simulink model "Eem_StMac_Prj"  (R2013b)
settings: Solver=FixedStepDiscrete  StartTime=0.0  StopTime=inf  FixedStep=0.001  RelTol=1e-3
PreLoadFcn:
  | load('Eem_StMac_Sim_DataSpec.mat')
model workspace (MAT data in the model file):
  java : class17 (value not decoded)
  MCOS : class17 (value not decoded)
undefined symbols (not defined in the file): process, ProcessTrigger_Lib
libraries: Variable_Lib x21, Efx_Library x17, Parameter_Lib x16, DSM_Library x9, DeltaTime_Lib x2, SYC_Library x1, DGS_Misc_Lib x1
(part 2 of 2)

== stateflow chart Eem_StMac_Prj/Eem_StMac/Component_Functionality/Proc_10ms/EemStrtupShdwn_SF ==
  note: Eem_stAct shows present state for simulation
  state Init_Mode
    state Eem_stAct_1
      entry:
      Eem_stAct = 1; ...
      Eem_tiStEx = 0;
      //***********************************
      Eem_stDesBms = 0; ...
      Eem_stDesPt = 1; ...
      Eem_stDesDcdc = 0; ...
      //***********************************
  note: Waiting for Transition from Car, Startup Demand from "above"
  note: Startwish by driver
  state Init_Mode_BattOn_BRMOn
    state Eem_stAct_5
      entry:
      Eem_stAct = 5; ...
      //***********************************
      // nothing to do
      // waiting BRM/battery ECUs to be switched on
      //***********************************
  note: power on: batttery ECU and BRM ECU
  note: Batt pre run test finished and
      | BRM inittest with 14 V ready and
      | DCDC preruntest finished
  state Startup_Mode
    during:
    Eem_tiStEx=Eem_tiStEx +dT;
    note: Battery, BRM, DCDC: be ready for PreCharge !
    state Eem_stAct_10
      entry:
      Eem_tiStEx =0;
      //***********************************
      // no change
      //***********************************
      Eem_stAct =10;
      note: Start Initialisation
    note: Battery, BRM, DCDC are ready for PreCharge
    note: Init of all components finished,
        | voltage level for successful  PreCharge
        | is reached
    note: Init of all components finished,
        | voltage level for successful  PreCharge
        | is reached
    note: Precharge with DCDC-converter
    state Eem_stAct_16
      entry:
      //*************************************
      Eem_stDesBms = 5; ...
      //**************************************
      Eem_stAct = 16;
      note: Init finished
    state Eem_stAct_14
      entry:
      //*****************************
      Eem_stDesDcdc = 3; ...
      //*****************************
      Eem_stAct = 14;
    note: PreCharge with Battery
    state Eem_stAct_12
      entry:
      //******************************
      Eem_stDesBms = 3; ...
      //****************************
      Eem_stAct = 12;
    note: PreCharge finished
        |  => Battery has to close main relais
    note: Mainrelais is closed
    state Eem_stAct_20
      entry:
      //**********************************
      Eem_stDesPt = 5; ...
      Eem_stDesDcdc = 5; ...
      //*********************************
      Eem_stAct = 20;
      note: Idle requested
    note: components in idle
    state Eem_stAct_30
      entry:
      //**********************************
      Eem_stDesPt = 6; ....
      //*********************************
      Eem_stAct = 30;
      note: PTr be boss
    (default) -> Eem_stAct_10
    (junction 153) -> Eem_stAct_14 [order 1] : [PRECOPT_SC ==0]
    Eem_stAct_10 -> (junction 153)
    (junction 153) -> Eem_stAct_12 [order 2] : [PRECOPT_SC >=1]
    Eem_stAct_12 -> Eem_stAct_16 : [Mvb_stOperModAct == 4 && ...
        | abs(Mvb_uAct - Dcdc_uMvAct) < Eem_uDifPtdPrec_C && ...
        | abs(Mvb_uAct - ElM_uAct) < Eem_uDifPtdPrec_C && ...
        | abs(Mvb_iAct) < Eem_iMinNcsryCntctr_C ]
    Eem_stAct_14 -> Eem_stAct_16 : [Dcdc_stOperModAct == 3 && ...
        | abs(Mvb_uAct - Dcdc_uMvAct) < Eem_uDifPtdPrec_C && ...
        | abs(Mvb_uAct - ElM_uAct) < Eem_uDifPtdPrec_C && ...
        | abs(Dcdc_iMvAct) < Eem_iMinNcsryCntctr_C]
    Eem_stAct_16 -> Eem_stAct_20 : [Mvb_stOperModAct == 5]
    Eem_stAct_20 -> Eem_stAct_30 : [ElM_stOperModAct == 5 && ...
        |  Dcdc_stOperModAct == 5 ]
  note: Pre Charging and closing of battery connectors
  state Service Modes [group]
    note: Not yet used
  note: BRM has taken over control
  state Normal_Mode
    entry:
    Eem_tiStEx=0;
    (history)
    note: PTr has torque control
    note: BRS-Normal Operation mode
        | with DCDC in forward mode
    note: BRS-Normal Operation mode
        | with DCDC in reverse mode
    note: no BRM start
    note: BRM start
    state Eem_stAct_46
      entry:
      //*****************************
      Eem_stDesDcdc = 8;
      //*****************************
      Eem_stAct = 46;
      note: no ICE-start with BRM ->
          | start with 12-V-starter
    state Eem_stAct_47
      entry:
      //***************************
      Eem_stDesDcdc = 9;
      //****************************
      Eem_stAct = 47;
      note: ICE-start with BRM
    (default) -> Eem_stAct_46
    Eem_stAct_47 -> Eem_stAct_46 : [ElM_stOperModAct != 11]
    Eem_stAct_46 -> Eem_stAct_47 : [ElM_stOperModAct == 11]
  state Backup_Modes
    entry:
    Eem_tiStEx = 0;
    note: default transition leads to backupmode 600
    note: "Battery off"
    note: "Battery off with
        | communication loss"
    note: "Generator limitted"
    note: "BRM off"
    note: "DCDC off"
    note: "DCDC off with
        |  commincation loss"
    note: "all off after load reduction
    note: "Emergency off" (even under load)
    note: BRM works as Generator with limitted load
    note: BRM voltage controlled and DCDC in forwar,
        |  battery has to disconnect by itself
    note: shorttime switch off of Dcdc and BRM
    note: BRM, DCDC and battery off
    note: BRM voltagecontrolled,
        | DCDC in forward mode
    note: BRM off
    note: Switch off DCDC-Converter
    state Eem_stAct_196
      entry:
      //**************************
      Eem_stDesPt = 5; ...
      Eem_stDesDcdc = 5; ...
      //*************************
      Eem_stAct=196;
      during:
      Eem_tiStEx = Eem_tiStEx + dT;
    state Eem_stAct_700
      entry:
      //**************************
      Eem_stDesBms = 14; ...
      Eem_stDesPt = 13; ...
      Eem_stDesDcdc = 13; ...
      //***************************
      Eem_stAct=700;
    state Eem_stAct_550
      entry:
      //****************************
      //* nothing **/
      //*****************************
      Eem_stAct=550;
    state Eem_stAct_598
      entry:
      //****************************
      Eem_stDesPt = 5; ...
      Eem_stDesDcdc = 5; ...
      //*****************************
      Eem_stAct=598;
      during:
      Eem_tiStEx = Eem_tiStEx + dT;
    state Eem_stAct_300
      entry:
      //***********************
      Eem_stDesPt = 7; ...
      Eem_stDesDcdc = 8; ...
      //***********************
      Eem_stAct=300;
    state Eem_stAct_400
      entry:
      //************************
      Eem_stDesPt = 13; ...
      //************************
      Eem_stAct=400;
    state Eem_stAct_250
      entry:
      //**************************
      Eem_stDesPt = 7; ...
      Eem_stDesDcdc = 8; ...
      //*************************
      Eem_stAct=250;
    state Eem_stAct_500
      entry:
      //****************************
      Eem_stDesDcdc = 13; ...
      //*****************************
      Eem_stAct=500;
    note: condition for "no currentflow over battery contactors"
    note: !! fail save state !!
    note: condition for "no currentflow over battery contactors"
    state Eem_stAct_198
      entry:
      //*****************************
      Eem_stDesBms = 13; ...
      //*****************************
      Eem_stAct = 198;
      during:
      Eem_tiStEx = Eem_tiStEx + dT;
    note: disconnection of 48V battery
    state Eem_stAct_600
      entry:
      //*****************************
      Eem_stDesBms = 13; ...
      Eem_stDesPt = 13; ...
      Eem_stDesDcdc = 13; ...
      //*****************************
      Eem_stAct = 600;
    note: condition for "MV grid is down"
    state Eem_stAct_200
      entry:
      Eem_tiStEx =0 ;...
      //*****************************
      Eem_stDesPt = 7; ...
      Eem_stDesDcdc = 8; ...
      //****************************
      Eem_stAct = 200;
    note: BRM voltage controlled
        | DCDC in forward mode
    note: battery is disconnected
    (junction 545) -> Eem_stAct_700 [order 1] : [Eem_stDesBkup == 700]
    (default) -> (junction 545)
    (junction 545) -> Eem_stAct_598 [order 8]
    (junction 545) -> Eem_stAct_196 [order 5] : [Eem_stDesBkup == 200]
    (junction 545) -> Eem_stAct_550 [order 7] : [Eem_stDesBkup == 550]
    (junction 545) -> Eem_stAct_250 [order 6] : [Eem_stDesBkup == 250]
    (junction 545) -> Eem_stAct_500 [order 2] : [Eem_stDesBkup == 500]
    (junction 545) -> Eem_stAct_300 [order 4] : [Eem_stDesBkup == 300]
    (junction 545) -> Eem_stAct_400 [order 3] : [Eem_stDesBkup == 400]
    Eem_stAct_500 -> Eem_stAct_550 : [Eem_stDesBkup == 550]
    Eem_stAct_300 -> Eem_stAct_400 : [Eem_stDesBkup == 400]
    Eem_stAct_200 -> Eem_stAct_250 : [Eem_stDesBkup == 250]
    Eem_stAct_196 -> Eem_stAct_198 : [abs(ElM_iAct) < Eem_iMinNcsryCntctr_C && ...
        | abs(Dcdc_iMvAct)< Eem_iMinNcsryCntctr_C]
    Eem_stAct_598 -> Eem_stAct_600 : [abs(Mvb_iAct) < Eem_iMinNcsryCntctr_C]
    Eem_stAct_198 -> Eem_stAct_200 : [ElM_uAct < Eem_uMinNcsryPrec_C || ...
        | Dcdc_uMvAct <Eem_uMinNcsryPrec_C]
  state Temporary_Restriction_Mode
    during:
    //************************************
    Eem_stAct = Eem_stDesBkup;
    //************************************
  note: Temporary restriction by voltageproblems in MV grid
  note: Degraded Modes (failure)
  note: Normal Operation Mode
  state Normal_Shutdown_Mode
    state Eem_stAct_82
      entry:
      Eem_tiStEx = 0; ...
      //* keep postrun alive ***//
      Eem_flgShDwnXPostDrv = 1; ...
      //*******************************
      Eem_stDesPt = 5; ...
      Eem_stDesDcdc = 5; ...
      //*******************************
      Eem_stAct = 82;
      during:
      Eem_tiStEx = Eem_tiStEx+dT;
    note: idle demand to BRM and converter
    note: (BRM and converter in idle and) no currentflow at battery
    state Eem_stAct_85
      entry:
      //****************************
      Eem_stDesBms = 13; ...
      //*****************************
      Eem_stAct = 85;
      during:
      Eem_tiStEx = Eem_tiStEx+dT;
    note: Disconnection of 48V-Battery
    note: 48V-Battery says "disconnected" and
        | voltage is low
    state Eem_stAct_90
      entry:
      //****************************
      Eem_stDesPt = 13; ...
      Eem_stDesDcdc = 13; ...
      //****************************
      Eem_stAct = 90;
      note: battery is disconnected
    note: relais open and voltage off and BRM and converter off
    note: ignition off
    (default) -> Eem_stAct_82
    Eem_stAct_82 -> Eem_stAct_85 : [abs(Mvb_iAct) < Eem_iMinNcsryCntctr_C ]
    Eem_stAct_85 -> state51 : [ElM_uAct < Eem_uMinNcsryPrec_C || ...
        | Dcdc_uMvAct < Eem_uMinNcsryPrec_C]
  state Backup_Shutdown_Mode
    entry:
    Eem_tiStEx = 0;
    note: default transition leads to backupmode 600
    note: "Battery off"
    note: "Battery off with
        | communication loss"
    note: "Generator limitted"
    note: "BRM off"
    note: "DCDC off"
    note: "DCDC off with
        |  commincation loss"
    note: "all off after load reduction
    note: "Emergency off" (even under load)
    note: switch off of Dcdc and BRM
    note: switch off of Dcdc and BRM
    note: BRM, DCDC and battery off
    note: BRM voltagecontrolled, no
        | communication to BRM
    note: BRM off
    note: DCDC-Converter of, no communication
    note: DCDC-Converter of with communication
    state Eem_stAct_252
      entry:
      //* keep postrun alive ***//
      Eem_flgShDwnXPostDrv = 1; ...
      //**************************
      //* battery not listening **//
      Eem_stDesPt = 13; ...
      Eem_stDesDcdc = 13; ...
      //*************************
      Eem_stAct=252;
      during:
      Eem_tiStEx = Eem_tiStEx + dT;
    state Eem_stAct_202
      entry:
      //* keep postrun alive ***//
      Eem_flgShDwnXPostDrv = 1; ...
      //**************************
      Eem_stDesPt = 13; ...
      Eem_stDesDcdc = 13; ...
      //*************************
      Eem_stAct=202;
      during:
      Eem_tiStEx = Eem_tiStEx + dT;
    state Eem_stAct_602
      entry:
      //* keep postrun alive ***//
      Eem_flgShDwnXPostDrv = 1; ...
      //****************************
      //* nothing **/
      //*****************************
      Eem_stAct=602;
    state Eem_stAct_702
      entry:
      //* keep postrun alive ***//
      Eem_flgShDwnXPostDrv = 1; ...
      //**************************
      //** nothing **//
      //***************************
      Eem_stAct=702;
    state Eem_stAct_302
      entry:
      //* keep postrun alive ***//
      Eem_flgShDwnXPostDrv = 1; ...
      //***********************
      //* Pt not listening ***//
      Eem_stDesDcdc = 5; ...
      //***********************
      Eem_stAct=302;
      during:
      Eem_tiStEx = Eem_tiStEx + dT;
    state Eem_stAct_552
      entry:
      //* keep postrun alive ***//
      Eem_flgShDwnXPostDrv = 1; ...
      //****************************
      Eem_stDesPt = 5; ...
      //* Dcdc not listening **//
      //*****************************
      Eem_stAct=552;
      during:
      Eem_tiStEx = Eem_tiStEx + dT;
    state Eem_stAct_402
      entry:
      //* keep postrun alive ***//
      Eem_flgShDwnXPostDrv = 1; ...
      //************************
      Eem_stDesPt = 5; ...
      Eem_stDesDcdc = 5; ...
      //************************
      Eem_stAct=402;
      during:
      Eem_tiStEx = Eem_tiStEx + dT;
    state Eem_stAct_502
      entry:
      //* keep postrun alive ***//
      Eem_flgShDwnXPostDrv = 1; ...
      //****************************
      Eem_stDesPt = 5;...
      Eem_stDesDcdc = 5; ...
      //*****************************
      Eem_stAct=502;
      during:
      Eem_tiStEx = Eem_tiStEx + dT;
    note: !! fail save states !!
    note: condition for "no currentflow over battery contactors"
    note: condition for "no currentflow over battery contactors"
    state Eem_stAct_304
      entry:
      //*****************************
      Eem_stDesBms = 13; ...
      //*****************************
      Eem_stAct = 304;
      during:
      Eem_tiStEx = Eem_tiStEx + dT;
    state Eem_stAct_504
      entry:
      //*****************************
      Eem_stDesBms = 13; ...
      //*****************************
      Eem_stAct = 504;
      during:
      Eem_tiStEx = Eem_tiStEx + dT;
    note: battery disconnect
    note: condition for "MV grid is down"
    note: condition for "MV grid is down"
    note: condition for "MV grid is down"
    note: condition for "MV grid is down"
    (junction 630) -> Eem_stAct_702 [order 1] : [Eem_stAct == 700]
    (default) -> (junction 630)
    (junction 630) -> Eem_stAct_602 [order 8]
    (junction 630) -> Eem_stAct_202 [order 5] : [Eem_stAct == 200]
    (junction 630) -> Eem_stAct_552 [order 7] : [Eem_stAct == 550]
    (junction 630) -> Eem_stAct_252 [order 6] : [Eem_stAct == 250]
    (junction 630) -> Eem_stAct_502 [order 2] : [Eem_stAct == 500]
    (junction 630) -> Eem_stAct_302 [order 4] : [Eem_stAct == 300]
    (junction 630) -> Eem_stAct_402 [order 3] : [Eem_stAct == 400]
    Eem_stAct_702 -> (junction 678)
    Eem_stAct_602 -> (junction 678)
    Eem_stAct_402 -> Eem_stAct_304 : [abs(Mvb_iAct) < Eem_iMinNcsryCntctr_C]
    Eem_stAct_202 -> (junction 678) : [ElM_uAct < Eem_uMinNcsryPrec_C || ...
        | Dcdc_uMvAct <Eem_uMinNcsryPrec_C]
    Eem_stAct_302 -> Eem_stAct_304 : [abs(Mvb_iAct) < Eem_iMinNcsryCntctr_C]
    Eem_stAct_252 -> (junction 678) : [ElM_uAct < Eem_uMinNcsryPrec_C || ...
        | Dcdc_uMvAct <Eem_uMinNcsryPrec_C]
    Eem_stAct_502 -> Eem_stAct_504 : [abs(Mvb_iAct) < Eem_iMinNcsryCntctr_C]
    Eem_stAct_552 -> Eem_stAct_504 : [abs(Mvb_iAct) < Eem_iMinNcsryCntctr_C]
    Eem_stAct_304 -> (junction 678) : [Dcdc_uMvAct <Eem_uMinNcsryPrec_C]
    Eem_stAct_504 -> (junction 678) : [ElM_uAct < Eem_uMinNcsryPrec_C]
  note: Shutdown with "ignition off" from backup modes
  note: Shutdown with "ignition off"
  state Shut_Down_Mode_BattOff_BRMOff
    state Eem_stAct_777
      entry:
      Eem_tiStEx = 0; ...
      //**************************
      Eem_stDesBms = 14; ...
      Eem_stDesPt = 13; ...
      Eem_stDesDcdc = 13; ...
      //***************************
      Eem_stAct=777;
      during:
      Eem_tiStEx = Eem_tiStEx+dT;
    (default) -> Eem_stAct_777
  note: power off: batttery ECU and BRM ECU
  note: waiting time: give Batt and BRM chance to be switched off
  state All_Comp_Off_Mode
    state Eem_stAct_888
      entry:
      //* postrun may finish ***//
      Eem_flgShDwnXPostDrv = 0; ...
      Eem_tiStEx = 0; ...
      //**************************
      // nothing to do
      //***************************
      Eem_stAct=888;
    (default) -> Eem_stAct_888
  note: All components off, MV grid down
  (default) -> Init_Mode
  (junction 610) -> Init_Mode : [T15_st!=0]
  Init_Mode -> Init_Mode_BattOn_BRMOn : [T15_st != 0]
  Init_Mode_BattOn_BRMOn -> Normal_Shutdown_Mode [order 2] : [T15_st==0]
  Init_Mode_BattOn_BRMOn -> Startup_Mode [order 1] : [Mvb_stOperModAct == 2 && ...
      | ElM_stOperModAct == 1 && ...
      | Dcdc_stOperModAct == 2]
  Startup_Mode -> ? [order 3] : [Eem_stDesBackup >=200]
  Startup_Mode -> Backup_Modes [order 2] : [Eem_stDesBkup >=200]
  Startup_Mode -> Normal_Shutdown_Mode [order 3] : [Eem_tiStEx >= Eem_tiToutStEx_C&& ...
      | Eem_flgTmrDisbl==0]
  Startup_Mode -> Normal_Shutdown_Mode [order 1] : [T15_st==0]
  (junction 697) -> Backup_Modes [order 1] : [(Eem_stDesBkup==700|| ...
      | Eem_stDesBkup==600) && ...
      |  Eem_stAct!= 600 && ...
      |  (T15_st != 0)]
  Normal_Mode -> Temporary_Restriction_Mode [order 3] : [Eem_stDesBkup == 102 || ...
      | Eem_stDesBkup == 104 || ...
      | Eem_stDesBkup == 106 || ...
      | Eem_stDesBkup == 108]
  Normal_Mode -> Normal_Shutdown_Mode [order 1] : [T15_st==0]
  Normal_Mode -> Backup_Modes [order 2] : [Eem_stDesBkup >=200]
  Temporary_Restriction_Mode -> Normal_Mode [order 2] : [Eem_stDesBkup <= 100 || ...
      | Eem_stDesBkup >= 200]
  Backup_Modes -> (junction 697) [order 1] : [Eem_stAct!=196 && ...
      | Eem_stAct!=198 && ...
      | Eem_stAct!=598]
  Backup_Modes -> Backup_Shutdown_Mode [order 2] : [Eem_tiStEx >= Eem_tiToutStEx_C&& ...
      | Eem_flgTmrDisbl==0]
  Temporary_Restriction_Mode -> Normal_Shutdown_Mode [order 1] : [T15_st==0]
  (junction 697) -> Backup_Shutdown_Mode [order 2] : [T15_st == 0]
  Backup_Shutdown_Mode -> Shut_Down_Mode_BattOff_BRMOff : [Eem_tiStEx >= Eem_tiToutStEx_C&& ...
      | Eem_flgTmrDisbl==0]
  Normal_Shutdown_Mode -> Shut_Down_Mode_BattOff_BRMOff : [Eem_tiStEx >= Eem_tiToutStEx_C&& ...
      | Eem_flgTmrDisbl==0]
  Eem_stAct_30 -> Normal_Mode
  Shut_Down_Mode_BattOff_BRMOff -> (junction 610) [order 2] : [T15_st!=0]
  All_Comp_Off_Mode -> (junction 610) : [T15_st!=0]
  Shut_Down_Mode_BattOff_BRMOff -> All_Comp_Off_Mode [order 1] : [Eem_tiStEx>= Eem_tiWaitPwrSplyOff_C]
  (junction 678) -> Shut_Down_Mode_BattOff_BRMOff : [T15_st == 0]
  state51 -> Shut_Down_Mode_BattOff_BRMOff : [T15_st == 0]
  data: Eem_stAct output OneToOne_U16; Eem_stDesBms output OneToOne_U8; Eem_stDesPt output OneToOne_U8; Eem_stDesDcdc output OneToOne_U8; T15_st input boolean; Mvb_stOperModAct input OneToOne_U8; ElM_stOperModAct input OneToOne_U8; Dcdc_stOperModAct input OneToOne_U8; Mvl_stOperModAct input OneToOne_U8; Mvb_uAct input spg_q0p0039_S16; ElM_uAct input spg_q0p0039_S16; Dcdc_uMvAct input spg_q0p0039_S16; Mvl_uActMean input spg_q0p0039_S16; Mvb_iAct input Curr_A_q0p03125_COMPU_S16; ElM_iAct input Curr_A_q0p03125_COMPU_S16; Dcdc_iMvAct input Curr_A_q0p03125_COMPU_S16; Mvl_iActSum input Curr_A_q0p03125_COMPU_S16; PRECOPT_SC input OneToOne_U8; Eem_tiStEx output RBPtCel_ti_0p01_1_U16; Eem_iMinNcsryCntctr_C input Curr_A_q0p03125_COMPU_S16; Eem_uDifPtdPrec_C input spg_q0p0039_S16; Eem_uMinNcsryPrec_C input spg_q0p0039_S16; Eem_tiToutStEx_C input RBPtCel_ti_0p01_1_U16; Eem_tiWaitPwrSplyOff_C input RBPtCel_ti_0p01_1_U16; Eem_flgShDwnXPostDrv output boolean; Eem_stDesBkup input OneToOne_U16; MvGrid_u input spg_q0p0039_S16; Eem_flgTmrDisbl input boolean; dT input t_q0p000001_s_S32
